simulink model "Cv_05_Problem_2"  (R2022b)
settings: Solver=VariableStepAuto  StartTime=0.0  StopTime=100  MaxStep=0.01  MinStep=0.001  RelTol=1e-3
libraries: slpidlib x1
settings Model: Creator=honza  LastModifiedBy=honza

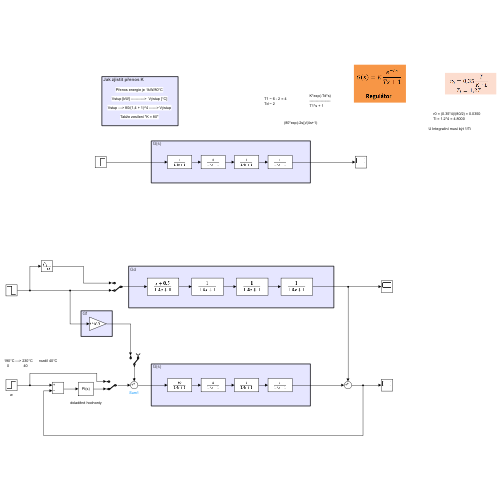
[thumbnail: Simulink's stored preview of the top-level diagram]
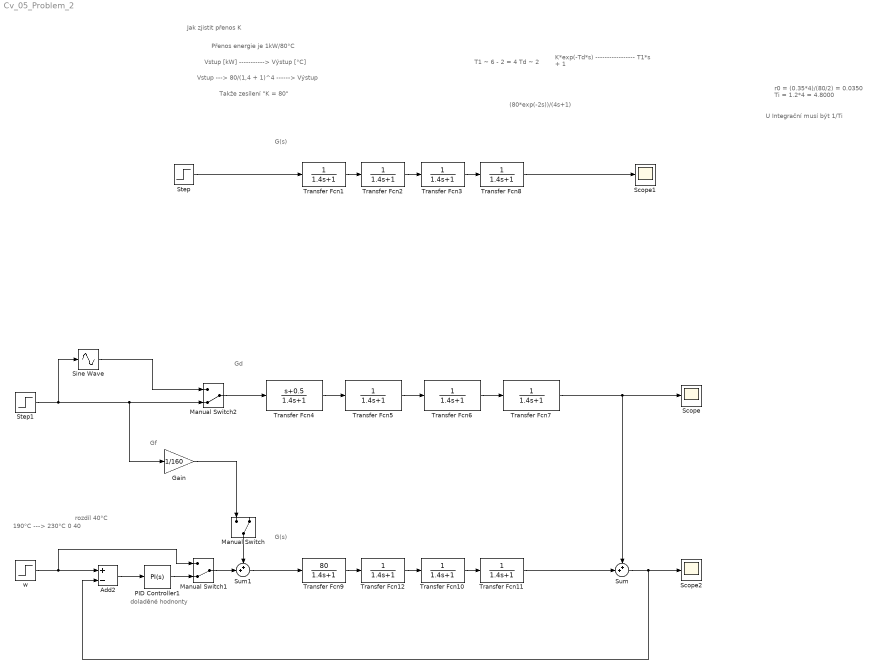
== system Cv_05_Problem_2 ==
  note: Gf
  note: Gd
  note: Vstup ---> 80/(1,4 + 1)^4 ------> Výstup
  note: G(s)
  note: (80*exp(-2s))/(4s+1)
  note: U Integrační musí být 1/Ti
  note: r0 = (0.35*4)/(80/2) = 0.0350
      | Ti = 1.2*4 = 4.8000
  note: 190°C ---> 230°C
      |    0              40
  note: T1 ~ 6 - 2 = 4
      | Td ~ 2
  note: K*exp(-Td*s)
      | -----------------
      | T1*s + 1
  note: Jak zjistit přenos K
  note: Takže zesílení "K = 80"
  note: G(s)
  note: Přenos energie je 1kW/80°C
  note: doladěné hodnonty
  note: Vstup [kW] -----------> Výstup [°C]
  note: rozdíl 40°C
  Add2 : Sum  Inputs=+-
  Gain : Gain  Gain=1/160
  Manual Switch : ManualSwitch  CurrentSetting=0
  Manual Switch1 : ManualSwitch  CurrentSetting=0
  Manual Switch2 : ManualSwitch  CurrentSetting=0
  PID Controller1 : slpidlib/PID Controller  Controller=PI  Form=Ideal  TimeDomain=Continuous-time  UseExternalTs=off  SampleTime=-1  IntegratorMethod=Forward Euler  FilterMethod=Forward Euler  ControllerParametersSource=internal  P=0.0055  I=1/3  UseKiTs=off  D=0  N=100  UseFilter=on  TunerSelectOption=Transfer Function Based (PID Tuner App)  InitialConditionSource=internal  InitialConditionForIntegrator=0  InitialConditionForFilter=0  DifferentiatorICPrevScaledInput=0  ExternalReset=none  TrackingMode=off  Kt=1  LimitOutput=off  SatLimitsSource=internal  UpperSaturationLimit=inf  LowerSaturationLimit=-inf  LinearizeAsGain=on  AntiWindupMode=none  Kb=1  LimitIntegrator=off  UpperIntegratorSaturationLimit=inf  LowerIntegratorSaturationLimit=-inf  POutMin=[]  POutMax=[]  IOutMin=[]  IOutMax=[]  DOutMin=[]  DOutMax=[]  NOutMin=[]  NOutMax=[]  SumOutMin=[]  SumOutMax=[]  SaturationOutMin=[]  SaturationOutMax=[]  PParamMin=[]  PParamMax=[]  IParamMin=[]  IParamMax=[]  DParamMin=[]  DParamMax=[]  NParamMin=[]  NParamMax=[]  KbParamMin=[]  KbParamMax=[]  KtParamMin=[]  KtParamMax=[]  KbOutMin=[]  KbOutMax=[]  KtOutMin=[]  KtOutMax=[]  IntegratorOutMin=[]  IntegratorOutMax=[]  FilterOutMin=[]  FilterOutMax=[]  SumI1OutMin=[]  SumI1OutMax=[]  SumI2OutMin=[]  SumI2OutMax=[]  SumI3OutMin=[]  SumI3OutMax=[]  SumI4OutMin=[]  SumI4OutMax=[]  SumDOutMin=[]  SumDOutMax=[]  DifferentiatorOutMin=[]  DifferentiatorOutMax=[]  FilterDiffOutCoefMin=[]  FilterDiffOutCoefMax=[]  ReciprocalOutMin=[]  ReciprocalOutMax=[]  SumDenOutMin=[]  SumDenOutMax=[]  SumNumOutMin=[]  SumNumOutMax=[]  DivideOutMin=[]  DivideOutMax=[]  UdiffTsProdOutMin=[]  UdiffTsProdOutMax=[]  NTsProdOutMin=[]  NTsProdOutMax=[]  UintegralTsProdOutMin=[]  UintegralTsProdOutMax=[]  UngainTsProdOutMin=[]  UngainTsProdOutMax=[]  ClampingZeroOutDataTypeStr=Inherit: Inherit via back propagation  ClampingZeroOutMin=[]  ClampingZeroOutMax=[]  FilterDenConstantOutDataTypeStr=Inherit: Inherit via back propagation  FilterDenConstantOutMin=[]  FilterDenConstantOutMax=[]  PCopyOutDataTypeStr=Inherit: Inherit via back propagation  PCopyOutMin=[]  PCopyOutMax=[]  NCopyOutDataTypeStr=Inherit: Inherit via back propagation  NCopyOutMin=[]  NCopyOutMax=[]  IntegratorContinuousStateAttributes=''  IntegratorStateMustResolveToSignalObject=off  IntegratorRTWStateStorageClass=Auto  FilterContinuousStateAttributes=''  FilterStateMustResolveToSignalObject=off  FilterRTWStateStorageClass=Auto  ParallelPVariant=Passthrough  IdealPVariant=InternalParameters  IVariant=InternalParameters  DVariant=Disabled  IntegratorVariant=Continuous  SatVariant=Disabled  AWVariant=Passthrough  PCopyVariant=Disabled  TRVariant=Disabled  FdbkBlocksVariant=Forward  IdealPFdbkVariant=Disabled  SatFdbkVariant=Disabled  DerivativeFilterVariant=Disabled  NVariant=Disabled  NCopyVariant=Disabled_SignalSpec  FilterICVariant=Disabled  IntegratorICVariant=InternalICs  ExternalResetVariant=Disabled  TRSumVariant=Passthrough  SumFdbkVariant=Disabled  SumVariant=Sum_PI  TsampFilterVariant=InternalTs  TsampNgainVariant=Passthrough  TsampIntegralVariant=Passthrough  ExternalSaturationOutDataTypeStr=Inherit: Same as second input
  Scope : Scope
  Scope1 : Scope
  Scope2 : Scope
  Sine Wave : Sin  TimeSource=Use external signal  SampleTime=0
  Step : Step  Time=0  SampleTime=0
  Step1 : Step  Time=60  Before=10  After=0  SampleTime=0
  Sum : Sum  Inputs=++|
  Sum1 : Sum  Inputs=++|
  Transfer Fcn{1..3,5..8,10..12} (10 alike) : TransferFcn  Denominator=[1.4 1]
  Transfer Fcn4 : TransferFcn  Numerator=[1 0.5]  Denominator=[1.4 1]
  Transfer Fcn9 : TransferFcn  Numerator=[80]  Denominator=[1.4 1]
  w : Step  Time=0  After=40  SampleTime=0
  wires:
  Transfer Fcn4/1 -> Transfer Fcn5/1
  Transfer Fcn6/1 -> Transfer Fcn7/1
  Transfer Fcn5/1 -> Transfer Fcn6/1
  w/1 -> Add2/1, Manual Switch1/1
  Transfer Fcn3/1 -> Transfer Fcn8/1
  Transfer Fcn10/1 -> Transfer Fcn11/1
  Transfer Fcn9/1 -> Transfer Fcn12/1
  Add2/1 -> PID Controller1/1
  Transfer Fcn2/1 -> Transfer Fcn3/1
  Transfer Fcn1/1 -> Transfer Fcn2/1
  Transfer Fcn12/1 -> Transfer Fcn10/1
  PID Controller1/1 -> Manual Switch1/2
  Step/1 -> Transfer Fcn1/1
  Transfer Fcn8/1 -> Scope1/1
  Transfer Fcn11/1 -> Sum/2
  Sum/1 -> Scope2/1, Add2/2
  Transfer Fcn7/1 -> Scope/1, Sum/1
  Step1/1 -> Sine Wave/1, Manual Switch2/2, Gain/1
  Manual Switch1/1 -> Sum1/2
  Sum1/1 -> Transfer Fcn9/1
  Manual Switch/1 -> Sum1/1
  Gain/1 -> Manual Switch/1
  Manual Switch2/1 -> Transfer Fcn4/1
  Sine Wave/1 -> Manual Switch2/1
